simulink model "FIR_TDM_Stream_Ex1"  (R2024a)
settings: Solver=VariableStepAuto  StartTime=0.0  StopTime=5  RelTol=1e-3
InitFcn:
  | NumOf_TDM_Channels = 16;
  | SamplesPerChannel = 64;
  | FilterLength = 32;
  | f = dsp.Channelizer(NumOf_TDM_Channels,1,Specification="coefficients");
  | blowpass = firpm(FilterLength-1,[0 .2 .4 1],[1 1 0 0]);
  | N = length(blowpass)-1;
  | Fc = 0.4;
  | j = complex(0,1);
  | bbandpass = blowpass.*exp(j*Fc*pi*(0:N));
  | f.LowpassCoefficients = bbandpass;
  | f.freqz
  | filters = f.getFilters;
  | filters = round(filters, 14, TieBreaker="fromzero");
undefined symbols (not defined in the file or in its folder): Asymmetric, S, vsva2197, xcvc1902
libraries: aieUtilities x5, aieDSP x1, dspobslib x1, dspsrcs4 x1, vmcUtilities x1
settings Model: Creator=sdegala  LastModifiedBy=robg
settings RTWCC: GPUComputeCapability=3.5
settings ConfigComp: CovBoundaryAbsTol=1.0e-5

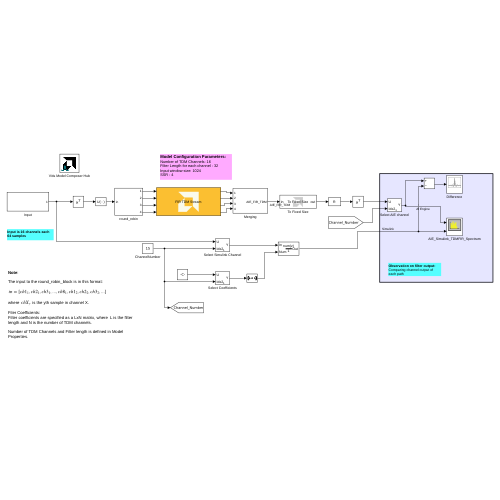
[thumbnail: Simulink's stored preview of the top-level diagram]
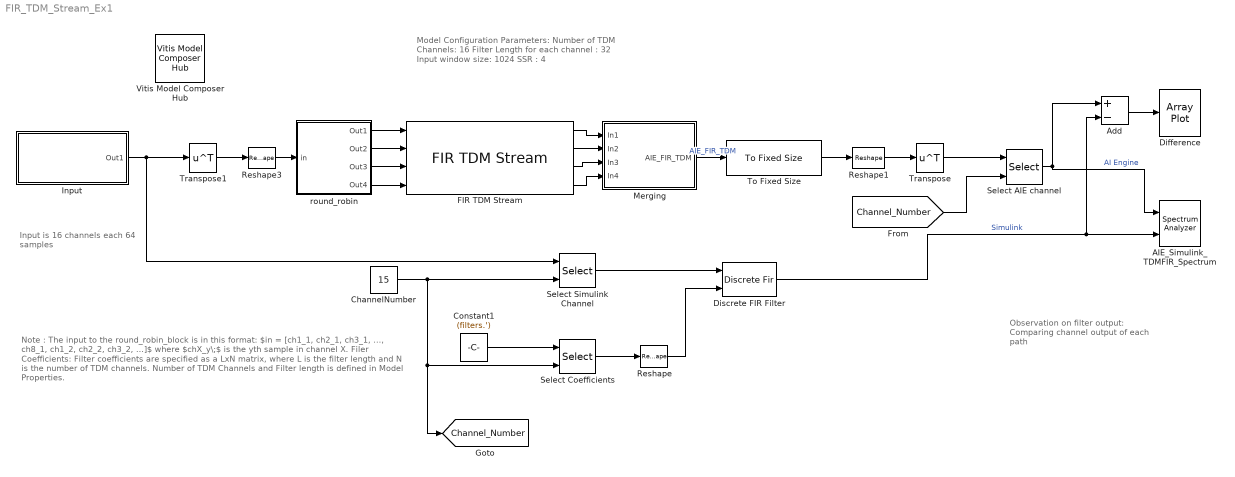
== system FIR_TDM_Stream_Ex1 ==
  note: Observation on filter output:
      | Comparing channel output of each path
  note: Input is 16 channels each 64 samples
  note: Model Configuration Parameters:
      | Number of TDM Channels: 16
      | Filter Length for each channel : 32
      | Input window size: 1024
      | SSR : 4
  note: Note :
      |
      | The input to the round_robin_block is in this format:
      |
      | $in = [ch1_1, ch2_1, ch3_1, ..., ch8_1, ch1_2, ch2_2, ch3_2, ...]$
      |
      | where $chX_y\;$ is the yth sample in channel X.
      |
      | Filer Coefficients:
      | Filter coefficients are specified as a LxN matrix, where L is the filter length and N is the number of TDM channels.
      |
      | Number of TDM Channels and Filter length is defined in Model Properties.
  AIE_Simulink_TDMFIR_Spectrum : SpectrumAnalyzer  NumInputPorts=2  WindowPosition=[247.000000,29.000000,936.000000,716.000000,]  Visible=on  ScopeFrameLocation=window  Span=12499.999999999998  StartFrequency=-6249.999999999999  StopFrequency=6249.999999999999  YLimits=[-89.98012941,-27.59367976]  ShowLegend=on  SelectedToolstripTab=spectrumAnalyzerToolstrip.channelMeasurementsTab  MeasurementChannel=2
  Add : Sum  Inputs=+-
  ChannelNumber : Constant  Value=15  OutDataTypeStr=uint16  SampleTime=-1
  Constant1 : Constant  Value=(filters.')  OutDataTypeStr=single  SampleTime=-1
  Difference : ArrayPlot  WindowPosition=[375.000000,26.000000,800.000000,500.000000,]  Visible=on  ScopeFrameLocation=window  XDataMode=Custom  XOffset=[-0.5 0.5]  PlotType=Line  AxesScaling=Manual  YLimits=[-0.5 0.5]  ShowLegend=on
  Discrete FIR Filter : DiscreteFir  CoefSource=Input port  Coefficients=filters(1,:)  InputProcessing=Columns as channels (frame based)  RndMeth=Round
      settings: InputPortMap=u0,u1
  FIR TDM Stream : aieDSP/FIR TDM Stream  data_type=cfloat  data_out_type=cfloat  use_coeff_reload=off  coef_type=cfloat  fir_length=FilterLength  coeff=(filters.')  shift_val=0  rnd_mode=Floor  input_window_size=SamplesPerChannel*NumOf_TDM_Channels  tdm_channels=NumOf_TDM_Channels  sat_mode=1-Asymmetric  casc_length=1  ssr=4  AIE_VARIANT=1  TP_API=0  dual_ip=0  TP_NUM_OUTPUTS=0  blockJsonConstraints=[]  blockJsonConstraintsInternal=[]  spec=vmc_stream_fir_tdm.json  SerializedMaskParamNames=[]  SerializedMaskParamValues=[]  SerializedMaskParamVisibilities=[]  block_type=FIR TDM Stream  SerializedMaskParamDataypes=typename|typename|uint|typename|uint|coef_type|uint|uint|uint|uint|uint|uint|uint|uint|uint|uint|uint  SerializedMaskParamEnumStrArr=0|0|0|0|0|0|0|Floor,Ceiling,Round to positive infinity,Round to negative infinity,Round symmetrical to infinity,Round symmetrical to zero,Round convergent to even,Round convergent to odd|0|0|0-None,1-Asymmetric,3-Symmetric|0|0|0|0|0|0  SerializedMaskParamEnumValArr=0|0|0|0|0|0|0|0,1,2,3,4,5,6,7|0|0|0,1,3|0|0|0|0|0|0  SerializedMaskParamVectorArr=0|0|0|0|0|1|0|0|0|0|0|0|0|0|0|0|0  SerializedMaskParamKeys=TT_DATA|TT_OUT_DATA|TP_USE_COEFF_RELOAD|TT_COEFF|TP_FIR_LEN|coeff|TP_SHIFT|TP_RND|TP_INPUT_WINDOW_VSIZE|TP_TDM_CHANNELS|TP_SAT|TP_CASC_LEN|TP_SSR|AIE_VARIANT|TP_API|TP_DUAL_IP|TP_NUM_OUTPUTS
  Input : Subsystem
  Merging : Subsystem
  Reshape : Reshape  OutputDimensionality=Row vector (2-D)
  Reshape1 : Reshape  OutputDimensionality=Customize  OutputDimensions=[NumOf_TDM_Channels,SamplesPerChannel]
  Reshape3 : Reshape
  Select AIE channel : Selector  NumberOfDimensions=2  InputPortWidth=3  IndexOptions=Select all,Index vector (port)  Indices=3,[16]  OutputSizes=1,1
  Select Coefficients : Selector  NumberOfDimensions=2  InputPortWidth=3  IndexOptions=Select all,Index vector (port)  Indices=3,[16]  OutputSizes=1,1
  Select Simulink Channel : Selector  NumberOfDimensions=2  InputPortWidth=3  IndexOptions=Select all,Index vector (port)  Indices=3,[16]  OutputSizes=1,1
  To Fixed Size : aieUtilities/To Fixed Size  Mode=Stop simulation when input variable-size signal is not full  OutputSize=Inherit: Same as input  CopyMethod=Buffer samples to form output  HasStatusOutput=on
  Transpose : Math  Operator=transpose
  Transpose1 : Math  Operator=transpose
  Vitis Model Composer Hub : vmcUtilities/Vitis Model Composer Hub  Tag=genX  CodeGeneration=off  StartColumn=1  NumberOfColumns=1  TargetDirectory=./code  exportDesign=off  analyzeDesign=off  validateDesignOnHw=off  ExportType=AI Engines  IpVendor=xilinx.com  IpLibrary=hls  IpVersion=1.0  IpHWLanguage=Verilog  AieCompilerOptions={}  AieSimulatorOptions={}  CreateTestbench=off  TestbenchStackSize=10  RunRtlSim=off  RunCSim=off  RunAieSim=off  AieSimTimeout=50000  RunAieSimProfiling=off  LaunchVitisAnalyzer=off  PlotOutput=off  RunX86Sim=off  X86SimTimeout=10  GenHwImage=off  GenLibadfXo=off  GenHwValidationCode=off  PlatformType=Not Specified  HwSystemType=Baremetal  HwValidationTarget=hw  ProjDevice=xcvc1902-vsva2197-1LP-e-S  ProjDevicePart=xcvc1902-vsva2197-1LP-e-S  AIEType=AIE  SamplePeriod=-1  ClockFrequency=200  DataPathParallelism=1  xilinxfamily=versalaicore  part=xcvc1902  speed=-1LP-e-S  package=vsva2197  directory=./netlist  testbench=off  incr_netlist=off  synthesis_tool=Vivado  clock_wrapper=Clock Enables  dbl_ovrd=According to Block Masks  dcm_input_clock_period=10  sysclk_period=10  simulink_period=1  eval_field=0  LogFileName=''  NThreads=4
  round_robin : Subsystem
  tag scope: Channel_Number=global
  wires:
  Reshape1/1 -> Transpose/1
  Select AIE channel/1 -> Add/1, AIE_Simulink_TDMFIR_Spectrum/1  "AI Engine"
  Transpose1/1 -> Reshape3/1
  Transpose/1 -> Select AIE channel/1
  Input/1(Out1) -> Transpose1/1, Select Simulink Channel/1
  Discrete FIR Filter/1 -> Add/2, AIE_Simulink_TDMFIR_Spectrum/2  "Simulink"
  Select Simulink Channel/1 -> Discrete FIR Filter/1
  Reshape3/1 -> round_robin/1(in)
  round_robin/1(Out1) -> FIR TDM Stream/1
  round_robin/2(Out2) -> FIR TDM Stream/2
  Merging/1(AIE_FIR_TDM) -> To Fixed Size/1  "AIE_FIR_TDM"
  FIR TDM Stream/1 -> Merging/1(In1)
  FIR TDM Stream/2 -> Merging/2(In2)
  round_robin/3(Out3) -> FIR TDM Stream/3
  round_robin/4(Out4) -> FIR TDM Stream/4
  FIR TDM Stream/3 -> Merging/3(In3)
  FIR TDM Stream/4 -> Merging/4(In4)
  To Fixed Size/1 -> Reshape1/1
  ChannelNumber/1 -> Select Coefficients/2, [Channel_Number], Select Simulink Channel/2
  [Channel_Number] -> Select AIE channel/2
  Add/1 -> Difference/1
  Constant1/1 -> Select Coefficients/1
  Select Coefficients/1 -> Reshape/1
  Reshape/1 -> Discrete FIR Filter/2

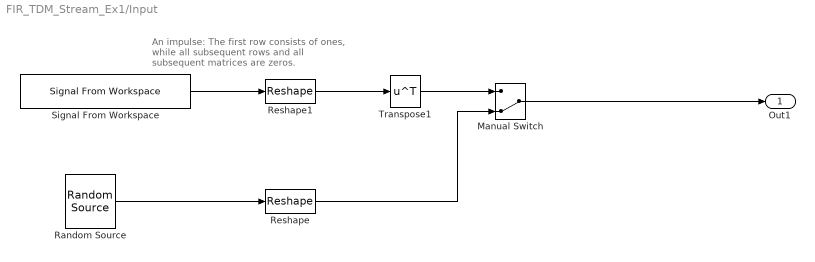
== system FIR_TDM_Stream_Ex1/Input ==
  note: An impulse: The first row consists of ones,
      | while all subsequent rows and all subsequent matrices are zeros.
  Manual Switch : ManualSwitch  CurrentSetting=0
  Random Source : dspobslib/Random Source  SrcType=Gaussian  NormMethod=Ziggurat  CltLength=12  MinVal=0  MaxVal=1  MeanVal=0  VarVal=1e-4  RepMode=Specify seed  rawSeed=1  IsInherit=off  SampMode=Discrete  SampTime=1/100e3  SampFrame=SamplesPerChannel*NumOf_TDM_Channels  DataType=Single  OutComplex=Complex  OutputFrames=on
  Reshape : Reshape  OutputDimensionality=Customize  OutputDimensions=[SamplesPerChannel,NumOf_TDM_Channels]
  Reshape1 : Reshape  OutputDimensionality=Customize  OutputDimensions=[NumOf_TDM_Channels,SamplesPerChannel]
  Signal From Workspace : dspsrcs4/Signal From Workspace  X=single(complex(ones(1,NumOf_TDM_Channels)))  Ts=1/100e3  nsamps=SamplesPerChannel*NumOf_TDM_Channels  OutputAfterFinalValue=Setting to zero  ignoreOrWarnInputAndFrameLengths=off  OutputFrames=off
  Transpose1 : Math  Operator=transpose
  Out1 : Outport
  wires:
  Manual Switch/1 -> Out1/1
  Random Source/1 -> Reshape/1
  Signal From Workspace/1 -> Reshape1/1
  Reshape/1 -> Manual Switch/2
  Reshape1/1 -> Transpose1/1
  Transpose1/1 -> Manual Switch/1

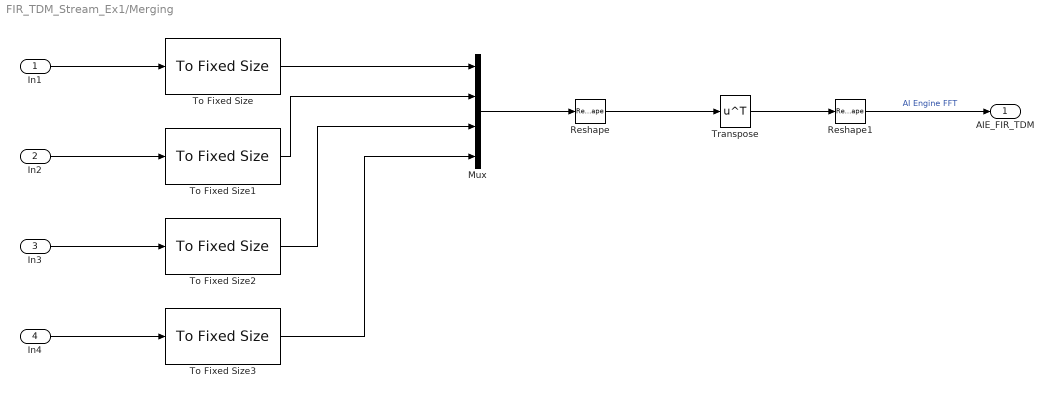
== system FIR_TDM_Stream_Ex1/Merging ==
  In1 : Inport
  In2 : Inport  Port=2
  In3 : Inport  Port=3
  In4 : Inport  Port=4
  Mux : Mux
  Reshape : Reshape  OutputDimensionality=Customize  OutputDimensions=[256, 4]
  Reshape1 : Reshape  OutputDimensions=[1, 10]
  To Fixed Size{,1..3} (4 alike) : aieUtilities/To Fixed Size  Mode=Stop simulation when input variable-size signal is not full  OutputSize=Inherit: Same as input  CopyMethod=Buffer samples to form output  HasStatusOutput=on
  Transpose : Math  Operator=transpose
  AIE_FIR_TDM : Outport
  wires:
  Reshape/1 -> Transpose/1
  To Fixed Size1/1 -> Mux/2
  In2/1 -> To Fixed Size1/1
  Transpose/1 -> Reshape1/1
  To Fixed Size/1 -> Mux/1
  Mux/1 -> Reshape/1
  Reshape1/1 -> AIE_FIR_TDM/1  "AI Engine FFT"
  In1/1 -> To Fixed Size/1
  To Fixed Size2/1 -> Mux/3
  In3/1 -> To Fixed Size2/1
  In4/1 -> To Fixed Size3/1
  To Fixed Size3/1 -> Mux/4

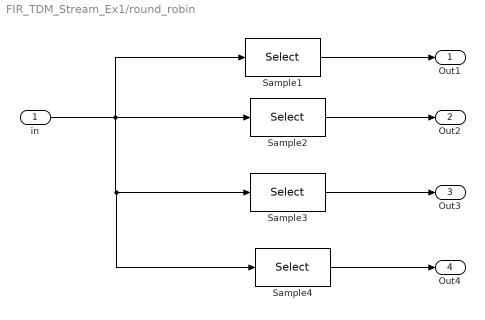
== system FIR_TDM_Stream_Ex1/round_robin ==
  in : Inport
  Sample1 : Selector  InputPortWidth=1024  IndexOptions=Index vector (dialog)  Indices=1:4:1024  OutputSizes=1
  Sample2 : Selector  InputPortWidth=1024  IndexOptions=Index vector (dialog)  Indices=2:4:1024  OutputSizes=1
  Sample3 : Selector  InputPortWidth=1024  IndexOptions=Index vector (dialog)  Indices=3:4:1024  OutputSizes=1
  Sample4 : Selector  InputPortWidth=1024  IndexOptions=Index vector (dialog)  Indices=4:4:1024  OutputSizes=1
  Out1 : Outport
  Out2 : Outport  Port=2
  Out3 : Outport  Port=3
  Out4 : Outport  Port=4
  wires:
  in/1 -> Sample4/1, Sample3/1, Sample2/1, Sample1/1
  Sample2/1 -> Out2/1
  Sample1/1 -> Out1/1
  Sample3/1 -> Out3/1
  Sample4/1 -> Out4/1
